simulink model "AeroWorkspaceTest1DOFStep"  (R2020a)
settings: Solver=ode1  StartTime=0.0  StopTime=30  FixedStep=0.002  RelTol=1e-3  EnableMultiTasking=on
undefined symbols (not defined in the file): HIL, qc_get_step_size
libraries: quarc_library x4
settings Model: ExtModeTrigDuration=5000  Creator=pmartin  LastModifiedBy=MLevis
settings DebuggingCC: UnderspecifiedInitializationDetection=Classic  MergeDetectMultiDrivingBlocksExec=none
settings ModelReferenceCC: PropagateSignalLabelsOutOfModel=off
settings SFSimCC: CustomCodeUndefinedFunction=UseInterfaceOnly
settings ExplorerConfigSet: SimMechanicsOpenEditorOnUpdate=off

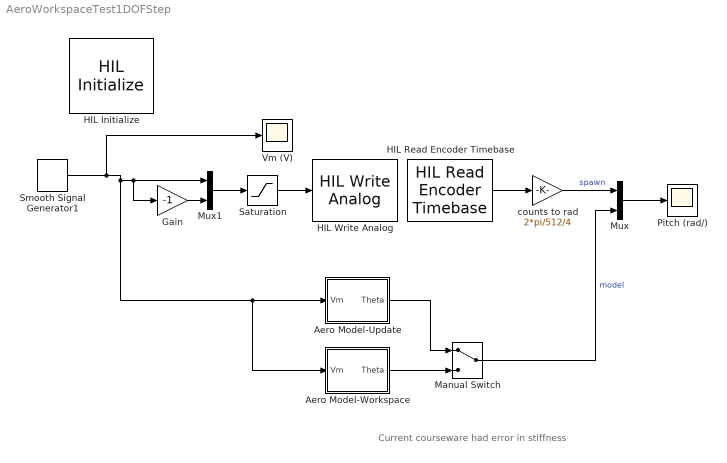
== system AeroWorkspaceTest1DOFStep ==
  note: Current courseware had error in stiffness
  Aero Model-Update : Subsystem
  Aero Model-Workspace : Subsystem
  Gain : Gain  Gain=-1
  HIL Initialize : quarc_library/Data Acquisition/Generic/Configuration/HIL Initialize  Priority=-99  object_name=HIL-1  board_type=quanser_aero_usb  board_number=0@tcpip://localhost:18930  board_options=""  exclusive=off  active=on  hardware_clocks=[0]  clock_modes=[]  initial_clock_frequencies=[]  set_clock_params_at_start=off  set_clock_params_at_switch_in=off  set_clock_frequencies_at_start=off  set_clock_frequencies_at_switch_in=off  analog_input_channels=[0:1]  analog_input_configurations=[]  analog_input_maximums=3  analog_input_minimums=-3  set_analog_input_params_at_start=off  set_analog_input_params_at_switch_in=off  analog_output_channels=[0:1]  analog_output_maximums=24  analog_output_minimums=-24  initial_analog_outputs=[0]  final_analog_outputs=[0]  watchdog_analog_outputs=[0]  set_analog_output_params_at_start=off  set_analog_output_params_at_switch_in=off  set_analog_outputs_at_start=on  set_analog_outputs_at_switch_in=off  set_analog_outputs_at_terminate=on  set_analog_outputs_at_switch_out=off  set_analog_outputs_on_watchdog=off  digital_input_channels=[]  digital_output_channels=[0:1]  digital_output_configuration=[]  initial_digital_outputs=[1]  final_digital_outputs=[0]  watchdog_digital_outputs=[0]  set_digital_output_params_at_start=off  set_digital_output_params_at_switch_in=off  set_digital_outputs_at_start=on  set_digital_outputs_at_switch_in=off  set_digital_outputs_at_terminate=on  set_digital_outputs_at_switch_out=off  set_digital_outputs_on_watchdog=off  encoder_channels=[0:3]  quadrature=[4]  encoder_filter_frequency=[]  initial_encoder_counts=[0]  set_encoder_params_at_start=off  set_encoder_params_at_switch_in=off  set_encoder_counts_at_start=on  set_encoder_counts_at_switch_in=off  pwm_channels=[]  pwm_modes=[]  pwm_frequency=[]  pwm_configuration=[]  pwm_alignment=[]  pwm_polarity=[]  pwm_leading_deadband=[]  pwm_trailing_deadband=[]  initial_pwm_outputs=[]  final_pwm_outputs=[]  watchdog_pwm_outputs=[]  set_pwm_params_at_start=off  set_pwm_params_at_switch_in=off  set_pwm_outputs_at_start=off  set_pwm_outputs_at_switch_in=off  set_pwm_outputs_at_terminate=off  set_pwm_outputs_at_switch_out=off  set_pwm_outputs_on_watchdog=off  other_output_channels=[11000:11002]  initial_other_outputs=[0 1 0]  final_other_outputs=[1 0 0]  watchdog_other_outputs=[0 0 1]  set_other_outputs_at_start=on  set_other_outputs_at_switch_in=off  set_other_outputs_at_terminate=on  set_other_outputs_at_switch_out=off  set_other_outputs_on_watchdog=off
  HIL Read Encoder Timebase : quarc_library/Data Acquisition/Generic/Timebases/HIL Read Encoder Timebase  object_name=HIL-1  clock=0  channels=2  active=on  vector_output=off  data_type_mode=Inherit via back propagation  data_type=double  overflow_mode=Synchronize (for simulated cards only)  samples_in_buffer=max(ceil(1/qc_get_step_size), 1)
  HIL Write Analog : quarc_library/Data Acquisition/Generic/Immediate I//O/HIL Write Analog  object_name=HIL-1  channels=[0:1]  sample_time=-1  active=on  vector_input=on
  Manual Switch : ManualSwitch
  Mux : Mux  Inputs=2
  Mux1 : Mux  Inputs=2
  Pitch (rad/) : Scope
  Saturation : Saturate  UpperLimit=24  LowerLimit=0
  Smooth Signal Generator1 : quarc_library/Sources/Signals/Smooth Signal Generator  signal_type=Square  source=Internal (dialog parameters)  amplitude=18  frequency=0.025  initial_phase=0  sample_time=qc_get_step_size  output_cos=off
      settings: SourceProductName=QUARC Targets
  Vm (V) : Scope
  counts to rad : Gain  Gain=2*pi/512/4
  wires:
  HIL Read Encoder Timebase/1 -> counts to rad/1
  counts to rad/1 -> Mux/1  "spawn"
  Mux/1 -> Pitch (rad/)/1
  Aero Model-Workspace/1(Theta) -> Manual Switch/2
  Aero Model-Update/1(Theta) -> Manual Switch/1
  Manual Switch/1 -> Mux/2  "model"
  Gain/1 -> Mux1/2
  Smooth Signal Generator1/1 -> Vm (V)/1, Aero Model-Workspace/1(Vm), Aero Model-Update/1(Vm), Gain/1, Mux1/1
  Mux1/1 -> Saturation/1
  Saturation/1 -> HIL Write Analog/1

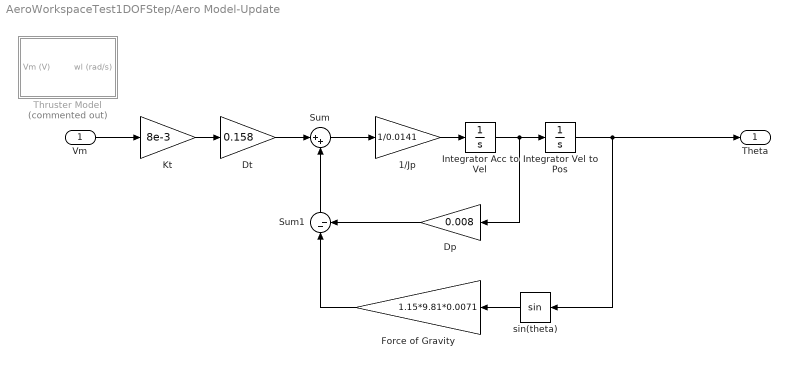
== system AeroWorkspaceTest1DOFStep/Aero Model-Update ==
  Vm : Inport
  1/Jp : Gain  Gain=1/0.0141
  Dp : Gain  Gain=0.008
  Dt : Gain  Gain=0.158
  Force of Gravity : Gain  Gain=1.15*9.81*0.0071
  Integrator Acc to Vel : Integrator
  Integrator Vel to Pos : Integrator
  Kt : Gain  Gain=8e-3
  Sum : Sum  Inputs=|++
  Sum1 : Sum  Inputs=|--
  Thruster Model : Subsystem  Commented=on
  "sin(theta) " : Trigonometry
  Theta : Outport
  wires:
  Sum/1 -> 1/Jp/1
  1/Jp/1 -> Integrator Acc to Vel/1
  Integrator Acc to Vel/1 -> Dp/1, Integrator Vel to Pos/1
  Dp/1 -> Sum1/2
  Sum1/1 -> Sum/2
  Kt/1 -> Dt/1
  Force of Gravity/1 -> Sum1/1
  "sin(theta) "/1 -> Force of Gravity/1
  Dt/1 -> Sum/1
  Integrator Vel to Pos/1 -> Theta/1, "sin(theta) "/1
  Vm/1 -> Kt/1

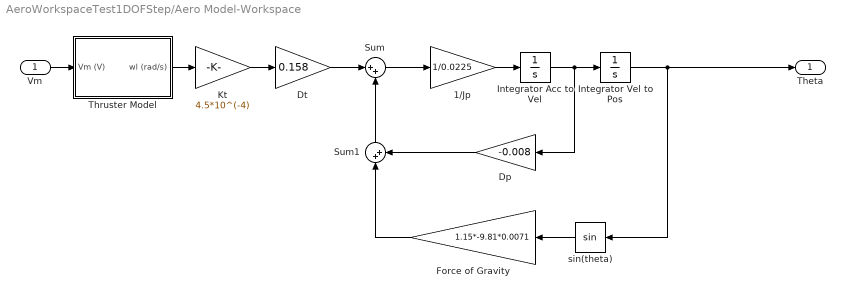
== system AeroWorkspaceTest1DOFStep/Aero Model-Workspace ==
  Vm : Inport
  1/Jp : Gain  Gain=1/0.0225
  Dp : Gain  Gain=-0.008
  Dt : Gain  Gain=0.158
  Force of Gravity : Gain  Gain=1.15*-9.81*0.0071
  Integrator Acc to Vel : Integrator
  Integrator Vel to Pos : Integrator
  Kt : Gain  Gain=4.5*10^(-4)
  Sum : Sum  Inputs=|++
  Sum1 : Sum  Inputs=|++
  Thruster Model : Subsystem
  "sin(theta) " : Trigonometry
  Theta : Outport
  wires:
  Vm/1 -> Thruster Model/1(Vm (V))
  Thruster Model/1(wl (rad/s)) -> Kt/1
  Integrator Vel to Pos/1 -> "sin(theta) "/1, Theta/1
  Dt/1 -> Sum/1
  "sin(theta) "/1 -> Force of Gravity/1
  Force of Gravity/1 -> Sum1/1
  Kt/1 -> Dt/1
  Sum1/1 -> Sum/2
  Dp/1 -> Sum1/2
  Integrator Acc to Vel/1 -> Integrator Vel to Pos/1, Dp/1
  1/Jp/1 -> Integrator Acc to Vel/1
  Sum/1 -> 1/Jp/1

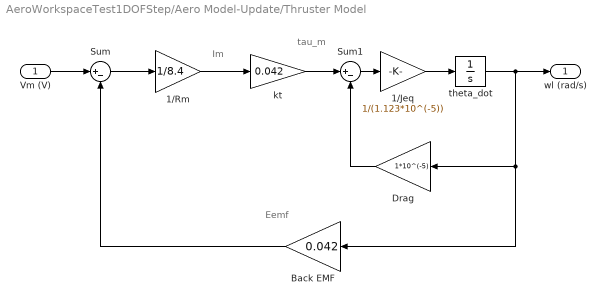
== system AeroWorkspaceTest1DOFStep/Aero Model-Update/Thruster Model ==
  note: Im
  note: tau_m
  note: Eemf
  Vm (V) : Inport
  1/Jeq : Gain  Gain=1/(1.123*10^(-5))  SaturateOnIntegerOverflow=on  OutDataTypeStr=Inherit: Same as input  ParamDataTypeStr=Inherit: Same as input
  1/Rm : Gain  Gain=1/8.4  SaturateOnIntegerOverflow=on  OutDataTypeStr=Inherit: Same as input  ParamDataTypeStr=Inherit: Same as input
  Back EMF : Gain  Gain=0.042  SaturateOnIntegerOverflow=on  OutDataTypeStr=Inherit: Same as input  ParamDataTypeStr=Inherit: Same as input
  Drag : Gain  Gain=1*10^(-5)  SaturateOnIntegerOverflow=on  OutDataTypeStr=Inherit: Same as input  ParamDataTypeStr=Inherit: Same as input
  Sum : Sum  Inputs=|+-  InputSameDT=on  SaturateOnIntegerOverflow=on  OutDataTypeStr=Inherit: Same as first input
  Sum1 : Sum  Inputs=|+-  InputSameDT=on  SaturateOnIntegerOverflow=on  OutDataTypeStr=Inherit: Same as first input
  kt : Gain  Gain=0.042
  theta_dot : Integrator
  wl (rad/s) : Outport
  wires:
  1/Rm/1 -> kt/1
  Vm (V)/1 -> Sum/1
  Sum/1 -> 1/Rm/1
  theta_dot/1 -> Back EMF/1, Drag/1, wl (rad/s)/1
  1/Jeq/1 -> theta_dot/1
  Back EMF/1 -> Sum/2
  kt/1 -> Sum1/1
  Sum1/1 -> 1/Jeq/1
  Drag/1 -> Sum1/2

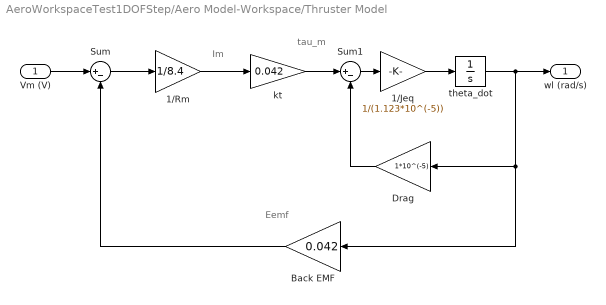
== system AeroWorkspaceTest1DOFStep/Aero Model-Workspace/Thruster Model ==
  note: Eemf
  note: tau_m
  note: Im
  Vm (V) : Inport
  1/Jeq : Gain  Gain=1/(1.123*10^(-5))  SaturateOnIntegerOverflow=on  OutDataTypeStr=Inherit: Same as input  ParamDataTypeStr=Inherit: Same as input
  1/Rm : Gain  Gain=1/8.4  SaturateOnIntegerOverflow=on  OutDataTypeStr=Inherit: Same as input  ParamDataTypeStr=Inherit: Same as input
  Back EMF : Gain  Gain=0.042  SaturateOnIntegerOverflow=on  OutDataTypeStr=Inherit: Same as input  ParamDataTypeStr=Inherit: Same as input
  Drag : Gain  Gain=1*10^(-5)  SaturateOnIntegerOverflow=on  OutDataTypeStr=Inherit: Same as input  ParamDataTypeStr=Inherit: Same as input
  Sum : Sum  Inputs=|+-  InputSameDT=on  SaturateOnIntegerOverflow=on  OutDataTypeStr=Inherit: Same as first input
  Sum1 : Sum  Inputs=|+-  InputSameDT=on  SaturateOnIntegerOverflow=on  OutDataTypeStr=Inherit: Same as first input
  kt : Gain  Gain=0.042
  theta_dot : Integrator
  wl (rad/s) : Outport
  wires:
  Drag/1 -> Sum1/2
  Sum1/1 -> 1/Jeq/1
  kt/1 -> Sum1/1
  Back EMF/1 -> Sum/2
  1/Jeq/1 -> theta_dot/1
  theta_dot/1 -> wl (rad/s)/1, Drag/1, Back EMF/1
  Sum/1 -> 1/Rm/1
  Vm (V)/1 -> Sum/1
  1/Rm/1 -> kt/1
